simulink model "bike_model"  (R2022b)
settings: Solver=FixedStepAuto  StartTime=0.0  StopTime=300  FixedStep=0.01  RelTol=1e-3
values from neighbouring files (symbols this model uses):
  gearboxRatio = 2412/187    (= 12.8983957219)    [veh_parameters.m]
  massTotal_kg = 310    [veh_parameters.m]
  wheelBaseRear_m = 0.6885    [veh_parameters.m]
  wheelRadius_m = 0.203    [veh_parameters.m]
libraries: autolibshared x2, simulink_extras x1
settings Model: Creator=LinF  LastModifiedBy=LinF
settings SolverCC: ConcurrentTasks=on  PositivePriorityOrder=on
settings OptimizationCC: BlockReduction=off  OptimizeBlockIOStorage=off
settings DebuggingCC: TasksWithSamePriorityMsg=none
settings HardwareCC: ProdBitPerLong=64  ProdLongLongMode=on  ProdHWDeviceType=Intel->x86-64 (Linux 64)
settings RTWCC: Description=Simulink Real-Time  SystemTargetFile=slrealtime.tlc  TemplateMakefile=slrealtime_default_tmf  Toolchain=Simulink Real-Time Toolchain  BuildConfiguration=Faster Runs  CodeExecutionProfiling=on  TargetLang=C++

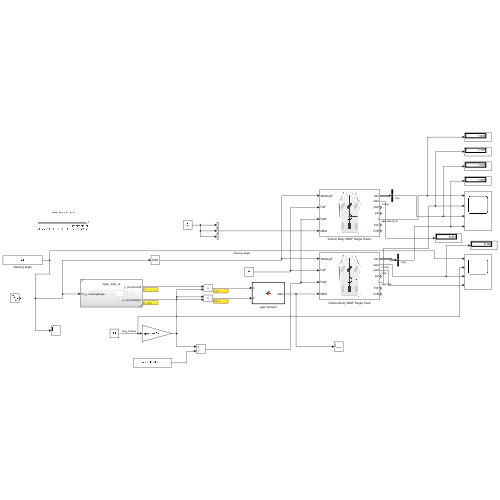
[thumbnail: Simulink's stored preview of the top-level diagram]
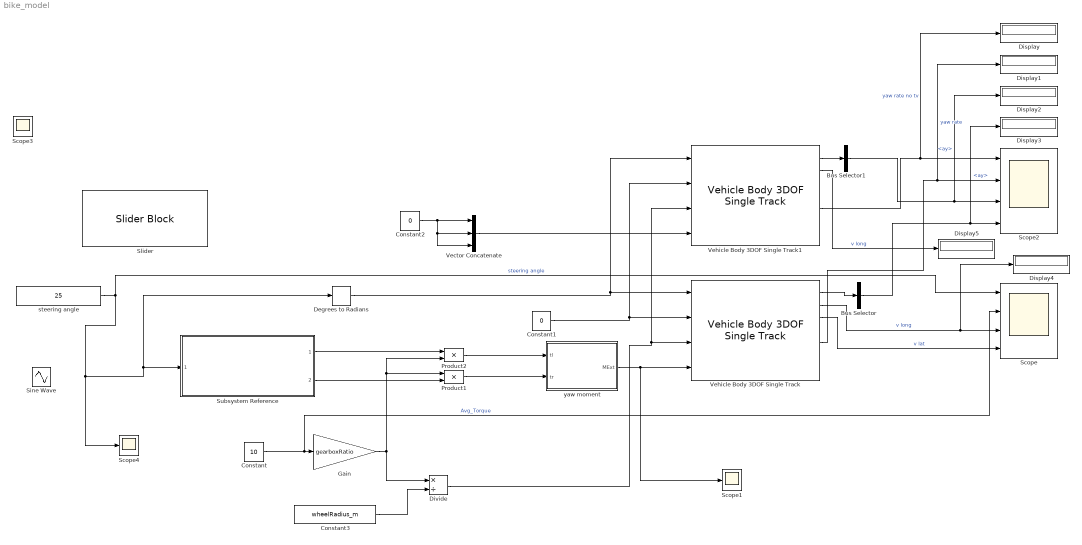
== system bike_model ==
  Bus Selector : BusSelector  OutputSignals=BdyFrm.Cg.Acc.ay
  Bus Selector1 : BusSelector  OutputSignals=BdyFrm.Cg.Acc.ay
  Constant : Constant  Value=10
  Constant1 : Constant  Value=0
  Constant2 : Constant  Value=0
  Constant3 : Constant  Value=wheelRadius_m
  Degrees to Radians : simulink_extras/Transformations/Degrees to Radians
  Display{,1..5} (6 alike) : Display
  Divide : Product  Inputs=*/
  Gain : Gain  Gain=gearboxRatio
  Product1 : Product
  Product2 : Product
  Scope : Scope  NumInputPorts=4
  Scope1 : Scope
  Scope2 : Scope  NumInputPorts=4
  Scope4 : Scope
  Sine Wave : Sin  Amplitude=25  SampleTime=0
  Slider : SliderBlock  ScaleMin=-25  ScaleMax=25
  Subsystem Reference : Subsystem  ReferencedSubsystem=open_loop_tv
  Vector Concatenate : Concatenate  NumInputs=3
  Vehicle Body 3DOF Single Track : autolibshared/Vehicle Body 3DOF Single Track  trackMode=Single (bicycle)  inputMode=External longitudinal forces  frontSteerMode=on  rearSteerMode=off  windMode=off  muMode=off  extFMode=off  extMMode=on  htchFMode=off  htchMMode=off  extXo=off  extpsio=off  extxdoto=off  extro=off  extYo=off  extTamb=off  extydoto=off  aMode=2  NF=2  NR=2  m=massTotal_kg  a=wheelBaseFront_m  b=wheelBaseRear_m  h=cgHeight_m  dh=1  hh=0.2  X_o=0  xdot_o=0  CalphaMode=off  sigmaMode=off  d=0  hl=0  w=[1.4,1.4]  Cy_f=CyFront_N_per_Rad  Cy_r=CyRear_N_per_Rad  sigma_f=.1  sigma_r=.1  alpha_f_brk=[-.1 .1]  Cy_f_data=[-9e3 9e3]  alpha_r_brk=[-.1 .1]  Cy_r_data=[-9e3 9e3]  Y_o=0  ydot_o=0  Izz=yawInertia_kg_per_mSqrd  psi_o=0  r_o=0  Af=dragArea_mSqrd  Cd=Cd  Cl=Cl  Cpm=.1  beta_w=[0 0.01:0.01:0.3]  Cs=[0 0.01:0.01:0.3]  Cym=[0 1e-6:0.01:0.3]  Pabs=101325  Tair=273  g=9.81  mu=1  xdot_tol=.01  Fznom=5000  Fxtire_sat=7e4  Fytire_sat=7e4  longOff=0  latOff=0  vertOff=0  wrapAng=off
  Vehicle Body 3DOF Single Track1 : autolibshared/Vehicle Body 3DOF Single Track  trackMode=Single (bicycle)  inputMode=External longitudinal forces  frontSteerMode=on  rearSteerMode=off  windMode=off  muMode=off  extFMode=off  extMMode=on  htchFMode=off  htchMMode=off  extXo=off  extpsio=off  extxdoto=off  extro=off  extYo=off  extTamb=off  extydoto=off  aMode=2  NF=2  NR=2  m=massTotal_kg  a=wheelBaseFront_m  b=wheelBaseRear_m  h=cgHeight_m  dh=1  hh=0.2  X_o=0  xdot_o=0  CalphaMode=off  sigmaMode=off  d=0  hl=0  w=[1.4,1.4]  Cy_f=CyFront_N_per_Rad  Cy_r=CyRear_N_per_Rad  sigma_f=.1  sigma_r=.1  alpha_f_brk=[-.1 .1]  Cy_f_data=[-9e3 9e3]  alpha_r_brk=[-.1 .1]  Cy_r_data=[-9e3 9e3]  Y_o=0  ydot_o=0  Izz=yawInertia_kg_per_mSqrd  psi_o=0  r_o=0  Af=dragArea_mSqrd  Cd=Cd  Cl=Cl  Cpm=.1  beta_w=[0 0.01:0.01:0.3]  Cs=[0 0.01:0.01:0.3]  Cym=[0 1e-6:0.01:0.3]  Pabs=101325  Tair=273  g=9.81  mu=1  xdot_tol=.01  Fznom=5000  Fxtire_sat=7e4  Fytire_sat=7e4  longOff=0  latOff=0  vertOff=0  wrapAng=off
  steering angle : Constant  Value=25
  yaw moment : MATLAB Function  TreatAsAtomicUnit=on
  Scope3 : Scope
  wires:
  Vehicle Body 3DOF Single Track/1 -> Bus Selector/1
  Vehicle Body 3DOF Single Track/3 -> Scope/4  "v lat"
  Vehicle Body 3DOF Single Track/2 -> Display4/1, Scope/3  "v long"
  Vehicle Body 3DOF Single Track/5 -> Scope2/2, Display1/1  "yaw rate"
  Constant/1 -> Scope/2, Gain/1  "Avg_Torque"
  Product2/1 -> yaw moment/1(tl)
  Product1/1 -> yaw moment/2(tr)
  Subsystem Reference/1 -> Product2/1
  Subsystem Reference/2 -> Product1/2
  Degrees to Radians/1 -> Vehicle Body 3DOF Single Track1/1, Vehicle Body 3DOF Single Track/1
  yaw moment/1(MExt) -> Scope1/1, Vehicle Body 3DOF Single Track/4
  steering angle/1 -> Scope/1, Scope4/1, Degrees to Radians/1, Subsystem Reference/1  "steering angle"
  Vector Concatenate/1 -> Vehicle Body 3DOF Single Track1/4
  Vehicle Body 3DOF Single Track1/5 -> Display/1, Scope2/1  "yaw rate no tv"
  Constant2/1 -> Vector Concatenate/3, Vector Concatenate/2, Vector Concatenate/1
  Constant1/1 -> Vehicle Body 3DOF Single Track1/2, Vehicle Body 3DOF Single Track/2
  Constant3/1 -> Divide/2
  Divide/1 -> Vehicle Body 3DOF Single Track1/3, Vehicle Body 3DOF Single Track/3
  Vehicle Body 3DOF Single Track1/1 -> Bus Selector1/1
  Bus Selector1/1 -> Scope2/3, Display2/1  "<ay>"
  Bus Selector/1 -> Display3/1, Scope2/4  "<ay>"
  Gain/1 -> Divide/1, Product2/2, Product1/1
  Vehicle Body 3DOF Single Track1/2 -> Display5/1  "v long"

== matlab function bike_model/yaw moment ==
  data: tl input; MExt output; tr input
function MExt = fcn(tl,tr)
m = (tl/0.203-tr/0.203)*0.5*1.285;
MExt = [0,0,m];
